simulink subsystem "attitude_determination_control_subsystem"  (R2023b)
settings: Solver=VariableStepAuto  StartTime=0.0  StopTime=10.0  RelTol=1e-3
settings Model: Creator=gio  LastModifiedBy=gio

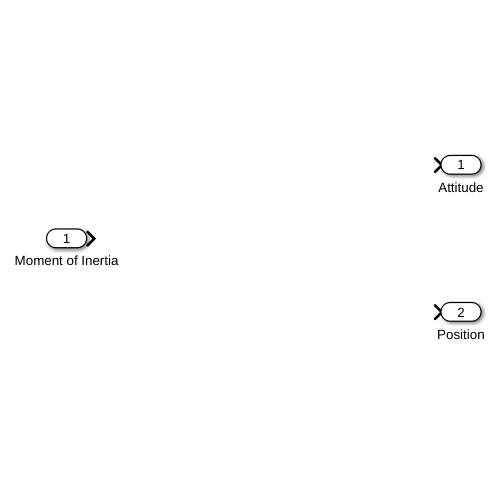
[thumbnail: Simulink's stored preview of the top-level diagram]
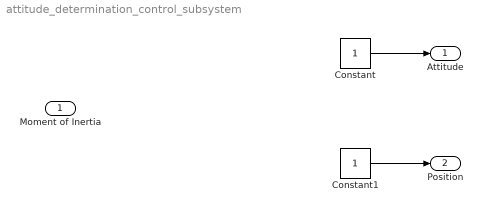
== system attitude_determination_control_subsystem ==
  Moment of Inertia : Inport
  Constant : Constant
  Constant1 : Constant
  Attitude : Outport
  Position : Outport  Port=2
  wires:
  Constant1/1 -> Position/1
  Constant/1 -> Attitude/1
